simulink model "state_space_all_andres"  (R2018a)
settings: Solver=ode8  StartTime=0.0  StopTime=10  FixedStep=tm  RelTol=1e-3
InitFcn:
  | A_SimulinkInit_linea_transmision
values from neighbouring files (symbols this model uses):
  b = 4.91    [SimulinkInit_linea_transmision.m]
  C = 1    [SimulinkInit_linea_transmision.m]
  C1 = 22e-6    (= 2.2e-05)    [SimulinkInit_linea_transmision.m]
  C2 = 22e-6    (= 2.2e-05)    [SimulinkInit_linea_transmision.m]
  C3 = 610e-6    (= 0.00061)    [SimulinkInit_linea_transmision.m]
  Cl = 20000e-6    (= 0.02)    [SimulinkInit_linea_transmision.m]
  Jd = 0.3    [SimulinkInit_linea_transmision.m]
  K = 25    [SimulinkInit_linea_transmision.m]    (also in uio_linear.m = K1+E*H)
  K1 = 9.66    [SimulinkInit_linea_transmision.m]    (also in uio_linear.m = K1')
  K11 = 0.8    [SimulinkInit_linea_transmision.m]
  K1d = 1.15    [SimulinkInit_linea_transmision.m]
  K2 = 6.97    [SimulinkInit_linea_transmision.m]
  K22 = 0.2    [SimulinkInit_linea_transmision.m]
  K2d = 1    [SimulinkInit_linea_transmision.m]
  K3 = 31.8    [SimulinkInit_linea_transmision.m]
  K33 = 0.23    [SimulinkInit_linea_transmision.m]
  K3d = 1    [SimulinkInit_linea_transmision.m]
  K4 = 15.1    [SimulinkInit_linea_transmision.m]
  Kd = 0.02    [SimulinkInit_linea_transmision.m]
  Kdc = 0.02    [SimulinkInit_linea_transmision.m]
  Kf = 1    [SimulinkInit_linea_transmision.m]
  Kh = 1.2    [SimulinkInit_linea_transmision.m]
  Ks = 21.5    [SimulinkInit_linea_transmision.m]
  Ksc = 3    [SimulinkInit_linea_transmision.m]
  Kv = 1    [SimulinkInit_linea_transmision.m]
  L = 5.2    [SimulinkInit_linea_transmision.m]
  L1 = 40e-3    (= 0.04)    [SimulinkInit_linea_transmision.m]
  L2 = 30e-3    (= 0.03)    [SimulinkInit_linea_transmision.m]
  L3 = 5e-3    (= 0.005)    [SimulinkInit_linea_transmision.m]
  L4 = 35e-6    (= 3.5e-05)    [SimulinkInit_linea_transmision.m]
  L5 = 22e-6    (= 2.2e-05)    [SimulinkInit_linea_transmision.m]
  L6 = 10e-6    (= 1e-05)    [SimulinkInit_linea_transmision.m]
  Pd = 0.1    [SimulinkInit_linea_transmision.m]
  R = 10    [SimulinkInit_linea_transmision.m]
  R1 = 0.1    [SimulinkInit_linea_transmision.m]
  R2 = 0.2    [SimulinkInit_linea_transmision.m]
  R3 = 1e-3    (= 0.001)    [SimulinkInit_linea_transmision.m]
  R4 = 0.005    [SimulinkInit_linea_transmision.m]
  R5 = 0.0012    [SimulinkInit_linea_transmision.m]
  R6 = 0.001    [SimulinkInit_linea_transmision.m]
  RL = 10    [SimulinkInit_linea_transmision.m]
  Sbin = 13.8    [SimulinkInit_linea_transmision.m]
  Svin = 2.91    [SimulinkInit_linea_transmision.m]
  T1 = 0.4    [SimulinkInit_linea_transmision.m]
  T2 = 1    [SimulinkInit_linea_transmision.m]
  T3 = 15    [SimulinkInit_linea_transmision.m]
  T4 = 2.5    [SimulinkInit_linea_transmision.m]
  Tao1d = 0.5    [SimulinkInit_linea_transmision.m]
  Tao2d = 0.125    [SimulinkInit_linea_transmision.m]
  Tcd = 0.2    [SimulinkInit_linea_transmision.m]
  Tcr = 0.01    [SimulinkInit_linea_transmision.m]
  Tf = 0.04    [SimulinkInit_linea_transmision.m]
  Tr = 950    [SimulinkInit_linea_transmision.m]
  Tt = 450    [SimulinkInit_linea_transmision.m]
  Ttd = 0.04    [SimulinkInit_linea_transmision.m]
  Tv = 0.05    [SimulinkInit_linea_transmision.m]
  V = 20    [SimulinkInit_linea_transmision.m]
  wref = 70000    [SimulinkInit_linea_transmision.m]
  X_acid = 1.2    [SimulinkInit_linea_transmision.m]
  X_meth = 0.35    [SimulinkInit_linea_transmision.m]
  Z = 3    [SimulinkInit_linea_transmision.m]
undefined symbols (not defined in the file or in its folder): Ad, Bd, C1o, C2o, C3o, C4o, Cd, F1, F2, F3, F4, H1, H2, H3, H4, K1U, K2U, K3U, K4U, T1s, T2s, T3s, T4s, T5s, tm
libraries: dsparch4 x4, powerlib_meascontrol x4, mpclib x1, simulink x1
(part 1 of 2)
settings Model: Creator=MarioAndres  LastModifiedBy=MarioAndres

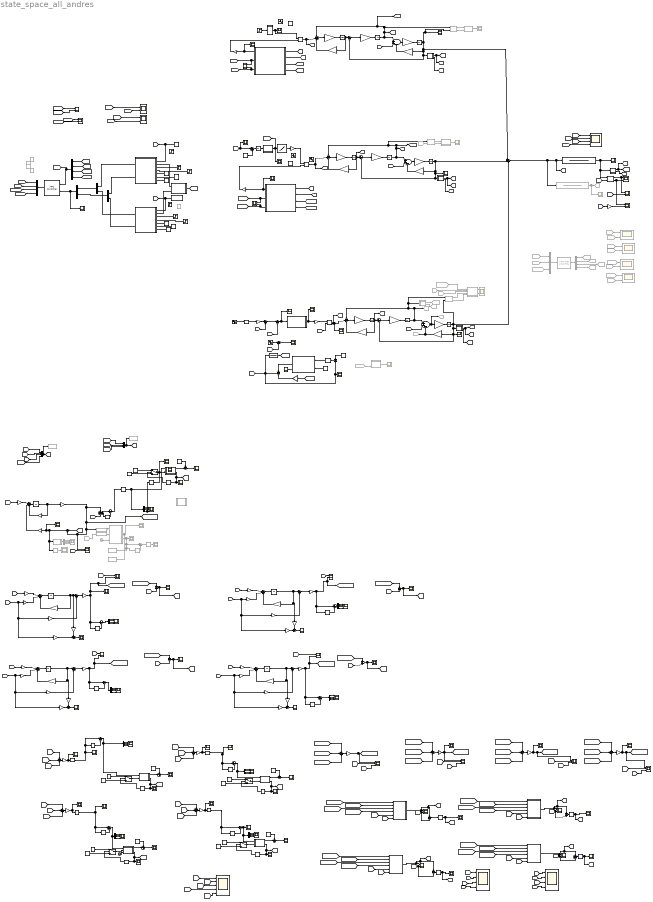
== system state_space_all_andres ==
  note: Nodo De Optimizacion
  note: CSI1-Biomasa
  note: CSI2-pv
  note: VSI-Diesel
  note: Carga RLC
  1-D Lookup Table2 : Lookup_n-D  NumberOfTableDimensions=1  BreakpointsForDimension1=[0 10 20 30 40 50 70 80 100]  Table=[0 10 200 500 800 1000 1140 1150 1200]  InternalRulePriority=Speed  RndMeth=Simplest  InputSameDT=on
  Abs{,1..3,5..9} (9 alike) : Abs
  Abs4 : Abs  Commented=on
  CSI_Control_BIO : Subsystem  mask{A=[0.0201   -0.039932     0.01986], B=[1     -1.9966       0.998], T=0.0001, st_time=0, Dn=[1     -1.0364], Dd=[1    -0.96364]}
      mask prompts: A "Numerador del control PR(z)"; B "Denominador del control PR(z)"; T "Tiempo de muestreo"; st_time "Tiempo_muerto"; Dn "Dn (Numerador de D(z))"; Dd "Dd (numerador de D(z))"
      mask DialogControl descripcion Prompt: Lazo de control de corriente para inversor monofasico. La entrada es un setpoint de potencia [P, Q]. Con ese setpoint se calcula la referencia de corriente sinusoidal deacuerdo a la tension medida de la red. Por lo anterior este controlador solo es valido para un inversor conectado a la red pues hara que se comporte como un CSI.
      mask DialogControl Control2 Prompt: Dn y Dd corresponden al numerador y denominador de la funcion de transferencia en Z (denominada D(z)) que hara un desfase de 90 de las señales medidas de tension y corriente del inversor. Estos desfases permiten mimificar las señales alfa y beta, de esta forma usar la misma teoria de potencia instantanea para el caso monofasico.
  CSI_Control_BIO1 : Subsystem  mask{A=[0.0201   -0.039932     0.01986], B=[1     -1.9966       0.998], T=0.0001, st_time=0, Dn=[1     -1.0364], Dd=[1    -0.96364]}
      mask prompts: A "Numerador del control PR(z)"; B "Denominador del control PR(z)"; T "Tiempo de muestreo"; st_time "Tiempo_muerto"; Dn "Dn (Numerador de D(z))"; Dd "Dd (numerador de D(z))"
      mask DialogControl descripcion Prompt: Lazo de control de corriente para inversor monofasico. La entrada es un setpoint de potencia [P, Q]. Con ese setpoint se calcula la referencia de corriente sinusoidal deacuerdo a la tension medida de la red. Por lo anterior este controlador solo es valido para un inversor conectado a la red pues hara que se comporte como un CSI.
      mask DialogControl Control2 Prompt: Dn y Dd corresponden al numerador y denominador de la funcion de transferencia en Z (denominada D(z)) que hara un desfase de 90 de las señales medidas de tension y corriente del inversor. Estos desfases permiten mimificar las señales alfa y beta, de esta forma usar la misma teoria de potencia instantanea para el caso monofasico.
  Clock1 : Clock  Commented=on
  Clock2 : Clock
  Constant : Constant  Commented=on  Value=-400
  Constant1 : Constant  Commented=on  Value=5000
  Constant{5..6,9..10,12,22..23,27..28,32} (10 alike) : Constant
  Constant11 : Constant  Value=1000
  Constant13 : Constant  Value=6000
  Constant14 : Constant  Value=5000
  Constant15 : Constant  Value=972.8
  Constant16 : Constant  Value=8000
  Constant17 : Constant  Value=115400
  Constant18 : Constant  Value=5000
  Constant19 : Constant  Value=8000
  Constant2 : Constant  Commented=on  Value=5000
  Constant20 : Constant  Value=10000
  Constant{7..8,21,24,31} (5 alike) : Constant  Value=0
  Constant25 : Constant  Value=1000
  Constant26 : Constant  Commented=on  Value=11210
  Constant29 : Constant  Value=1000
  Constant3 : Constant  Commented=on  Value=8000
  Constant30 : Constant  Value=0.1
  Control PR VSI1 : Subsystem
  Current Panel : Constant  Value=1.5
  Delay : Delay  DelayLength=1
  Demux : Demux  Commented=on
  Demux{1..4,9..14} (10 alike) : Demux
  Demux19 : Demux  Commented=on
  Derivative2 : Derivative  CoefficientInTFapproximation=0
  Derivative4 : Derivative  Commented=on  CoefficientInTFapproximation=0
  Diesel Generator2 : Subsystem
  From : From  Commented=on  GotoTag=i1model
  From14 : From  Commented=on  GotoTag=i1
  From15 : From  Commented=on  GotoTag=i2
  From24 : From  Commented=on  GotoTag=Vload
  From25 : From  Commented=on  GotoTag=i3
  From30 : From  Commented=on  GotoTag=u2
  From33 : From  Commented=on  GotoTag=u3
  From37 : From  Commented=on  GotoTag=Papadiel
  From38 : From  Commented=on  GotoTag=Paparente
  From39 : From  Commented=on  GotoTag=Q_ref
  From40 : From  Commented=on  GotoTag=P_ref
  From47 : From  Commented=on  GotoTag=i2
  From6 : From  Commented=on  GotoTag=i2model
  From60 : From  Commented=on  GotoTag=y_ma
  From7 : From  Commented=on  GotoTag=i3model
  From8 : From  Commented=on  GotoTag=Vloadm
  From9 : From  Commented=on  GotoTag=u1
  Gain : Gain  Gain=1/L1
  Gain1 : Gain  Gain=1/C1
  Gain10 : Gain  Gain=1/L3
  Gain11 : Gain  Gain=1/C3
  Gain12 : Gain  Gain=1/L6
  Gain13 : Gain  Gain=R6
  Gain14 : Gain  Gain=R3
  Gain{15..18} (4 alike) : Gain  Gain=2
  Gain19 : Gain  Gain=C3
  Gain2 : Gain  Gain=1/L4
  Gain20 : Gain  Gain=-1
  Gain21 : Gain  Gain=.5
  Gain{22..29} (8 alike) : Gain  Gain=1/3
  Gain3 : Gain  Gain=R4
  Gain4 : Gain  Gain=R1
  Gain5 : Gain  Gain=1/L2
  Gain6 : Gain  Gain=1/C2
  Gain7 : Gain  Gain=1/L5
  Gain8 : Gain  Gain=R5
  Gain9 : Gain  Gain=R2
  Goto : Goto  Commented=on  GotoTag=i1model
  Goto1 : Goto  Commented=on  GotoTag=Vload
  Goto15 : Goto  Commented=on  GotoTag=i2model
  Goto16 : Goto  Commented=on  GotoTag=i3model
  Goto17 : Goto  Commented=on  GotoTag=v3
  Goto18 : Goto  Commented=on  GotoTag=vl6
  Goto19 : Goto  Commented=on  GotoTag=vr6
  Goto22 : Goto  Commented=on  GotoTag=Vloadm
  Goto61 : Goto  Commented=on  GotoTag=V_vsi
  Goto62 : Goto  Commented=on  GotoTag=a4
  Integrator{,1..8} (9 alike) : Integrator
  Integrator9 : Integrator  LimitOutput=on  UpperSaturationLimit=1  LowerSaturationLimit=0
  LinearProg2 : MATLAB Function  TreatAsAtomicUnit=on  SystemSampleTime=1e-3
  LinearProg3 : MATLAB Function  TreatAsAtomicUnit=on  SystemSampleTime=1e-3
  MATLAB Funcionando sin Vload conectado despues del ataque : MATLAB Function  Commented=on  TreatAsAtomicUnit=on
  "MATLAB Function SOC " : MATLAB Function  TreatAsAtomicUnit=on
  MATLAB Function1 : MATLAB Function  TreatAsAtomicUnit=on
  MATLAB Function12 : MATLAB Function  TreatAsAtomicUnit=on
  MATLAB Function13 : MATLAB Function  TreatAsAtomicUnit=on
  MATLAB Function17 : MATLAB Function  TreatAsAtomicUnit=on
  MATLAB Function18 : MATLAB Function  TreatAsAtomicUnit=on
  MATLAB Function2 : MATLAB Function  TreatAsAtomicUnit=on
  MATLAB Function3 : MATLAB Function  Commented=on  TreatAsAtomicUnit=on
  MATLAB Function34 : MATLAB Function  TreatAsAtomicUnit=on
  MATLAB Function36 : MATLAB Function  TreatAsAtomicUnit=on
  MATLAB Function38 : MATLAB Function  TreatAsAtomicUnit=on
  MATLAB Function39 : MATLAB Function  TreatAsAtomicUnit=on
  MATLAB Function4 : MATLAB Function  Commented=on  TreatAsAtomicUnit=on
  MATLAB Function5 : MATLAB Function  Commented=on  TreatAsAtomicUnit=on
  MATLAB Function6 : MATLAB Function  Commented=on  TreatAsAtomicUnit=on
  MATLAB Function7 : MATLAB Function  Commented=on  TreatAsAtomicUnit=on
  MATLAB Function8 : MATLAB Function  Commented=on  TreatAsAtomicUnit=on
  MPC Controller : mpclib/MPC Controller  SCDEnableBlockLinearizationSpecification=on  mpcobj=mpcobj  is_multiple=0  enable_value=0  return_u0=off  updateMPCinCallerWorkspace=on  ref_from_ws=off  ref_signal_name=[]  ref_preview=off  md_from_ws=off  md_signal_name=[]  md_preview=off  from_project=off  project_file=MPCtask.mat  md_inport=off  mv_inport=off  cost_outport=off  return_sequence=off  return_qpstatus=off  return_state=off  state_inport=off  lims_inport=off  cc_inport=off  ywt_inport=off  is_designfromscratch=0  uwt_inport=off  duwt_inport=off  rhoeps_inport=off  uref_inport=off  n_ts=0.1  n_p=100  n_mv=4  n_md=0  n_ud=0  n_mo=4  n_uo=0  BlockDataType=double  SampleTimeInherited=off  switch_inport=off
  MeasureNode_I1 : Subsystem
  MeasureNode_I2 : Subsystem
  MeasureNode_I3 : Subsystem
  MeasureNode_I4 : Subsystem
  MeasureNode_I5 : Subsystem  Commented=on
  Memory{,1..13} (14 alike) : Memory
  Memory14 : Memory  Commented=on
  Mux2 : Mux  Commented=on  Inputs=3
  Mux3 : Mux  Inputs=2
  Mux4 : Mux
  Mux5 : Mux  Inputs=2
  Mux6 : Mux  Inputs=2
  Mux7 : Mux  Inputs=3
  Mux8 : Mux
  PID Controller2 : simulink/Continuous/PID Controller  Controller=PID  TimeDomain=Continuous-time  SampleTime=-1  IntegratorMethod=Forward Euler  FilterMethod=Forward Euler  Form=Parallel  UseFilter=on  ControllerParametersSource=internal  P=0.000853612192208084  I=3.94394231511782e-05  D=0.00224356290205903  N=0.155980576752107  InitialConditionSource=internal  InitialConditionForIntegrator=0  InitialConditionForFilter=0  ExternalReset=none  LimitOutput=off  UpperSaturationLimit=inf  LowerSaturationLimit=-inf  LinearizeAsGain=on  AntiWindupMode=none  Kb=1  TrackingMode=off  Kt=1  PParamMin=[]  PParamMax=[]  IParamMin=[]  IParamMax=[]  DParamMin=[]  DParamMax=[]  NParamMin=[]  NParamMax=[]  KbParamMin=[]  KbParamMax=[]  KtParamMin=[]  KtParamMax=[]  POutMin=[]  POutMax=[]  IOutMin=[]  IOutMax=[]  DOutMin=[]  DOutMax=[]  NOutMin=[]  NOutMax=[]  KbOutMin=[]  KbOutMax=[]  KtOutMin=[]  KtOutMax=[]  IntegratorOutMin=[]  IntegratorOutMax=[]  FilterOutMin=[]  FilterOutMax=[]  SumOutMin=[]  SumOutMax=[]  SumI1OutMin=[]  SumI1OutMax=[]  SumI2OutMin=[]  SumI2OutMax=[]  SumI3OutMin=[]  SumI3OutMax=[]  SumDOutMin=[]  SumDOutMax=[]  SaturationOutMin=[]  SaturationOutMax=[]  IntegratorContinuousStateAttributes=''  IntegratorStateMustResolveToSignalObject=off  IntegratorRTWStateStorageClass=Auto  FilterContinuousStateAttributes=''  FilterStateMustResolveToSignalObject=off  FilterRTWStateStorageClass=Auto  DifferentiatorICPrevScaledInput=0  DifferentiatorOutMin=[]  DifferentiatorOutMax=[]  InitialConditionSetting=State (most efficient)  FilterDiffOutCoefMin=[]  FilterDiffOutCoefMax=[]  SumDenOutMin=[]  SumDenOutMax=[]  SumNumOutMin=[]  SumNumOutMax=[]  ReciprocalOutMin=[]  ReciprocalOutMax=[]  DivideOutMin=[]  DivideOutMax=[]  TunerSelectOption=Transfer Function Based (PID Tuner App)
  Power : powerlib_meascontrol/Measurements/Power  Freq=60  Vinit=[1, 0]  Iinit=[1, 0]  Ts=0
      settings: SourceProductName=Simscape Power Systems
  Power1 : powerlib_meascontrol/Measurements/Power  Commented=on  Freq=60  Vinit=[1, 0]  Iinit=[1, 0]  Ts=0
      settings: SourceProductName=Simscape Power Systems
  Power3 : powerlib_meascontrol/Measurements/Power  Commented=on  Freq=60  Vinit=[1, 0]  Iinit=[1, 0]  Ts=0
      settings: SourceProductName=Simscape Power Systems
  Power4 : powerlib_meascontrol/Measurements/Power  Commented=on  Freq=60  Vinit=[1, 0]  Iinit=[1, 0]  Ts=0
      settings: SourceProductName=Simscape Power Systems
  Product : Product
  Product1 : Product
  Product3 : Product
  Scope{,1,3,7,35} (5 alike) : Scope  Commented=on  NumInputPorts=2
  Scope{8,10..12,14..18,21,52..53,58,86..89,109} (18 alike) : Scope  NumInputPorts=2
  Scope{2,4..6,13,19..20,24..32,34,37..38,41..49,51,55..57,61,63..73,75,91,110,112,114,118,120..121,135} (53 alike) : Scope
  Scope{59..60,62,138} (4 alike) : Scope  NumInputPorts=3
  Scope{9,22,36,39..40,50,74,139} (8 alike) : Scope  Commented=on
  Scope{23,33,76..83,85,90} (12 alike) : Scope  NumInputPorts=4
  Scope54 : Scope  Commented=on  NumInputPorts=4
  Scope84 : Scope  NumInputPorts=5
  Signal Specification : SignalSpecification  Commented=on  Dimensions=4
  Signal Specification1 : SignalSpecification  Commented=on  Dimensions=4
  Sine Wave1 : Sin  Amplitude=170  Frequency=2*pi*60  SampleTime=0
  Sine Wave2 : Sin  Frequency=2*pi/0.025  SampleTime=0
  Sine Wave3 : Sin  Frequency=2*pi/0.025  SampleTime=0
  Sine Wave4 : Sin  Amplitude=170  Frequency=2*pi*60  SampleTime=0
  Sine Wave5 : Sin  Amplitude=60  Frequency=2*pi*60  SampleTime=0
  State-Space : StateSpace  Commented=on  A=|  B=|  C=[zeros(1,3) 1 zeros(1,7); zeros(1,4) 1 zeros(1,6); zeros(1,5) 1 zeros(1,5);zeros(1,10) 1]  D=zeros(4,3);  InitialCondition=0
      A=|
      | [-R1/L1 zeros(1,6) -1/L1 zeros(1,3);
      |     0 -R2/L2 zeros(1,6) -1/L2 0 0;
      |     zeros(1,2) -R3/L3 zeros(1,6) -1/L3 0;
      |     zeros(1,3) -R4/L4 zeros(1,3) 1/L4 0 0 -1/L4;
      |     zeros(1,4) -R5/L5 zeros(1,3) 1/L5 0 -1/L5;
      |     zeros(1,5) -R6/L6 zeros(1,3) 1/L6 -1/L6;
      |     zeros(1,6) -R/L zeros(1,3) 1/L;
      |     1/C1 zeros(1,2) -1/C1 zeros(1,7);
      |     0 1/C2 0 0 -1/C2 zeros(1,6);
      |     0 0 1/C3 0 0 -1/C3 zeros(1,5);
      |     zeros(1,3) 1/Cl 1/Cl 1/Cl -1/Cl zeros(1,3) -1/(Cl*RL)]
      B=|
      | [1/L1 0 0;
      |    0 1/L2 0;
      |    0 0 1/L3;
      |    zeros(8,3)];
  Step : Step  Time=0  After=28  SampleTime=0
  Step1 : Step  Time=200  Before=1.2  After=.4  SampleTime=0
  Step10 : Step  Time=20  Before=115400  After=15400  SampleTime=0
  Step4 : Step  Time=200  Before=1  After=0.4  SampleTime=0
  Step5 : Step  Time=200  Before=1  SampleTime=0
  Step8 : Step  Time=200  Before=.7  SampleTime=0
  Step9 : Step  Time=20  Before=978  After=1400  SampleTime=0
  Sum{,4,7,11,17,20,24..26,30,36..37,39..40,43} (15 alike) : Sum  Inputs=|+-
  Sum1 : Sum  Inputs=|+--
  Sum{10,12,14,22,38,74} (6 alike) : Sum  Inputs=|++
  Sum{13,15..16,18,27,33,42,67,70,72..73} (11 alike) : Sum  Inputs=+-
  Sum{19,31..32,71} (4 alike) : Sum  Inputs=-+|
  Sum2 : Sum  Inputs=|+++
  Sum{21,23,49,75..76} (5 alike) : Sum  Inputs=|+++  SampleTime=tm
  Sum{28..29,34..35,53} (5 alike) : Sum  Inputs=+-|
  Sum3 : Sum  Inputs=-|+-
  Sum41 : Sum  Commented=on  Inputs=|+-
  Sum5 : Sum  Inputs=|+--
  Sum{58..61,77..80} (8 alike) : Sum  Inputs=+++
  Sum6 : Sum  Inputs=-|+-
  Sum8 : Sum  Inputs=|+--
  Sum9 : Sum  Inputs=-|+-
  Switch{,1..4} (5 alike) : Switch  Criteria=u2 > Threshold
  To Workspace : ToWorkspace  Commented=on  VariableName=det1  SampleTime=1e-4
  To Workspace1 : ToWorkspace  Commented=on  VariableName=norm1  SampleTime=1e-4
  To Workspace2 : ToWorkspace  Commented=on  VariableName=y_ma  SampleTime=1e-4
  To Workspace3 : ToWorkspace  Commented=on  VariableName=u_fs  SampleTime=1e-4
  Transfer Fcn1 : TransferFcn  Commented=on  Numerator=[R*RL*L 0]  Denominator=[Cl*RL*R*L (RL+R)*L R*RL]
  Transfer Fcn3 : TransferFcn  Numerator=[RL*L RL*R]  Denominator="[Cl*RL*L  (R*RL*Cl+L) RL+R]"
  Transfer Fcn4 : TransferFcn  Denominator=[1e-4 1]
  Unit Delay{1..2,6..7,10} (5 alike) : UnitDelay  SampleTime=tm
  adis1 : Gain  Gain=F3  Multiplication=Matrix(K*u) (u vector)  SampleTime=tm
  adis10 : Gain  Gain=Ld'  Multiplication=Matrix(K*u) (u vector)  SampleTime=tm
  adis11 : Gain  Gain=F1  Multiplication=Matrix(K*u) (u vector)  SampleTime=tm
  adis12 : Gain  Gain=F2  Multiplication=Matrix(K*u) (u vector)  SampleTime=tm
  adis2 : Gain  Gain=F4  Multiplication=Matrix(K*u) (u vector)  SampleTime=tm
  adis7 : Gain  Gain=Ad  Multiplication=Matrix(K*u) (u vector)  SampleTime=tm
  bdis1 : Gain  Gain=T3*Bd  Multiplication=Matrix(K*u) (u vector)  SampleTime=tm
  bdis10 : Gain  Gain=T2*Bd  Multiplication=Matrix(K*u) (u vector)  SampleTime=tm
  bdis11 : Gain  Gain=K2U  Multiplication=Matrix(K*u) (u vector)  SampleTime=tm
  bdis12 : Gain  Gain=H2  Multiplication=Matrix(K*u) (u vector)  SampleTime=tm
  bdis13 : Gain  Gain=eye(1)-C2o*H2  Multiplication=Matrix(K*u) (u vector)  SampleTime=tm
  bdis14 : Gain  Gain=eye(1)-C1o*H1  Multiplication=Matrix(K*u) (u vector)  SampleTime=tm
  bdis15 : Gain  Gain=C1o  Multiplication=Matrix(K*u) (u vector)  SampleTime=tm
  bdis16 : Gain  Gain=C2o  Multiplication=Matrix(K*u) (u vector)  SampleTime=tm
  bdis17 : Gain  Gain=T4*Bd  Multiplication=Matrix(K*u) (u vector)  SampleTime=tm
  bdis18 : Gain  Gain=K4U  Multiplication=Matrix(K*u) (u vector)  SampleTime=tm
  bdis19 : Gain  Gain=H4  Multiplication=Matrix(K*u) (u vector)  SampleTime=tm
  bdis2 : Gain  Gain=K3U  Multiplication=Matrix(K*u) (u vector)  SampleTime=tm
  bdis20 : Gain  Gain=eye(1)-C4o*H4  Multiplication=Matrix(K*u) (u vector)  SampleTime=tm
  bdis21 : Gain  Gain=C4o  Multiplication=Matrix(K*u) (u vector)  SampleTime=tm
  bdis3 : Gain  Gain=H3  Multiplication=Matrix(K*u) (u vector)  SampleTime=tm
  bdis4 : Gain  Gain=eye(1)-C3o*H3  Multiplication=Matrix(K*u) (u vector)  SampleTime=tm
  bdis5 : Gain  Gain=Bd  Multiplication=Matrix(K*u) (u vector)  SampleTime=tm
  bdis6 : Gain  Gain=C3o  Multiplication=Matrix(K*u) (u vector)  SampleTime=tm
  bdis7 : Gain  Gain=T1*Bd  Multiplication=Matrix(K*u) (u vector)  SampleTime=tm
  bdis8 : Gain  Gain=K1U  Multiplication=Matrix(K*u) (u vector)  SampleTime=tm
  bdis9 : Gain  Gain=H1  Multiplication=Matrix(K*u) (u vector)  SampleTime=tm
  cdis{1..5} (5 alike) : Gain  Gain=Cd  Multiplication=Matrix(K*u) (u vector)  SampleTime=tm
  generador biomasa : Subsystem
  wires:
  Gain/1 -> Integrator/1
  Integrator/1 -> Gain4/1, Sum/1
  Sum/1 -> Gain1/1
  Gain1/1 -> Integrator1/1
  Integrator1/1 -> [v1], [V_bio], Sum3/1, Power3/1, Sum1/1
  Sum1/1 -> Gain2/1
  Gain2/1 -> Integrator2/1
  Integrator2/1 -> Power3/2, Scope4/1, Sum2/1, MeasureNode_I2/1(in), Sum/2, Gain3/1
  Gain3/1 -> Sum1/3
  Sum3/1 -> Gain/1
  Gain4/1 -> Sum3/3
  Sum2/1 -> Transfer Fcn1/1, [I_load], Transfer Fcn3/1
  Transfer Fcn3/1 -> MeasureNode_I4/1(in), Power/1, Scope2/1
  [Vload] -> Sum1/2
  Integrator3/1 -> [ipi], Gain9/1, Sum4/1
  Gain5/1 -> Integrator3/1
  Gain6/1 -> Integrator4/1
  Gain8/1 -> Sum5/3
  Gain7/1 -> Integrator5/1
  [Vload] -> Sum5/2
  Gain9/1 -> Sum6/3
  Sum6/1 -> Gain5/1
  Sum5/1 -> Gain7/1
  Sum4/1 -> Gain6/1
  Integrator6/1 -> [i3m], Gain14/1, Sum7/1
  Gain10/1 -> Integrator6/1
  Gain11/1 -> Integrator7/1
  Integrator7/1 -> MeasureNode_I5/1(in), Power1/1, Sum9/1, Goto17/1, Sum8/1
  Gain13/1 -> Goto19/1, Sum8/3
  Gain12/1 -> Integrator8/1
  [Vload] -> Sum8/2
  Gain14/1 -> Sum9/3
  Sum9/1 -> Gain10/1
  Sum8/1 -> Goto18/1, Gain12/1
  Sum7/1 -> Gain11/1
  Integrator8/1 -> Power1/2, Sum2/3, MeasureNode_I3/1(in), Gain13/1, Scope6/1, Sum7/2
  Integrator5/1 -> Sum2/2, Scope5/1, MeasureNode_I1/1(in), Sum4/2, Gain8/1
  [I_load] -> Power/2
  Power/1 -> Scope11/1, Scope10/1
  Power/2 -> Scope12/1, Scope10/2
  [P_ref] -> Scope11/2
  CSI_Control_BIO/2(Q_measure) -> [Qo_bio], Scope14/1
  CSI_Control_BIO/3(P_measure) -> [Po_bio], Scope14/2
  Control PR VSI1/1(d) -> Gain17/1, Scope28/1
  Product3/1 -> [u3], Sum9/2, Scope29/1
  CSI_Control_BIO1/2(Q_measure) -> [Qo_diesel], Scope21/1
  CSI_Control_BIO1/3(P_measure) -> [Po_diesel], Scope21/2
  Integrator4/1 -> [v2], [V_die], Power4/1, Sum6/1, Sum5/1
  Current Panel/1 -> Sum14/2
  Sum14/1 -> Integrator9/1
  [ipi] -> Scope27/1, Sum14/1  "inductor I measured"
  "MATLAB Function SOC "/1(y) -> [SOC], Scope26/1, 1-D Lookup Table2/1  "soc"
  1-D Lookup Table2/1 -> Gain18/1  "battery Vdc"
  Integrator9/1 -> "MATLAB Function SOC "/1(u)
  Derivative2/1 -> Gain19/1
  Gain19/1 -> Sum12/1
  Sine Wave1/1 -> Derivative2/1  "ref voltage"
  Sum11/1 -> Control PR VSI1/1(Ierror), Scope19/1
  Sum12/1 -> Sum11/1
  [i3] -> Sum12/2
  [i3m] -> Sum11/2
  Product1/1 -> Sum6/2, [u2]
  Step5/1 -> LinearProg3/3(kb)
  Mux4/1 -> [Paparente], MPC Controller/1
  Constant13/1 -> LinearProg3/7(Q_e_alt_min)
  [Qo_bio] -> Mux4/2
  Mux3/1 -> Scope32/1, MPC Controller/2
  LinearProg2/2(Pdo) -> Mux6/1  "die"
  Mux6/1 -> Mux3/2
  [SOC] -> MATLAB Function2/1(SOC)
  MPC Controller/1 -> Demux3/1
  [Qo_diesel] -> Mux4/4
  Constant14/1 -> LinearProg3/6(QbMax)
  Constant18/1 -> LinearProg2/7(P_e_alt_min)
  Mux5/1 -> Mux3/1
  [Po_diesel] -> Mux4/3
  Step4/1 -> LinearProg2/4(kd)
  Step1/1 -> LinearProg2/3(kb)
  Constant19/1 -> LinearProg3/5(QdMax)
  MATLAB Function2/1(MaxP) -> LinearProg2/2(P_e_alt)
  Constant20/1 -> LinearProg2/6(PbMax)
  MATLAB Function2/2(MaxQ) -> LinearProg3/2(Q_e_alt)
  Step8/1 -> LinearProg3/4(kd)
  LinearProg3/2(Qdo) -> Mux6/2
  [Po_bio] -> Mux4/1
  LinearProg3/1(Qbo) -> Mux5/2
  Constant16/1 -> LinearProg2/5(PdMax)
  LinearProg2/1(Pbo) -> Mux5/1  "bio"
  [Pi_bio] -> Scope16/2
  [Po_bio] -> Scope16/1
  [Qi_bio] -> Scope15/2
  [Qo_bio] -> Scope15/1
  [Qo_diesel] -> Scope17/1
  [Po_diesel] -> Scope18/1
  [Pi_Diesel] -> Scope18/2
  [Qi_diesel] -> Scope17/2
  [V_vsi] -> Scope23/4
  [V_die] -> Scope23/3
  [V_bio] -> Scope23/2
  [Vload] -> Scope23/1
  generador biomasa/1(Vdc) -> Product/1, Scope24/1
  Step/1 -> generador biomasa/1(In1)
  [v2] -> CSI_Control_BIO1/1(V_measured)
  [i2] -> CSI_Control_BIO1/2(I_measured)
  [v1] -> CSI_Control_BIO/1(V_measured)
  [i1] -> CSI_Control_BIO/2(I_measured)
  Gain18/1 -> Product1/1
  Gain15/1 -> Product/2
  Product/1 -> [u1], Sum3/2
  Gain16/1 -> Product1/2
  [Pi_Diesel] -> CSI_Control_BIO1/3(P_ref)
  [Qi_diesel] -> CSI_Control_BIO1/4(Q_ref)
  Gain17/1 -> Product3/1
  [Pi_bio] -> CSI_Control_BIO/3(P_ref)
  [Qi_bio] -> CSI_Control_BIO/4(Q_ref)
  [Q_ref] -> Gain20/1
  Gain20/1 -> Scope12/2
  MATLAB Function3/1(y) -> Scope22/1
  From37/1 -> MATLAB Function3/3(potencia)
  From38/1 -> MATLAB Function4/1(u)
  From40/1 -> MATLAB Function4/2(pref)
  From39/1 -> MATLAB Function4/3(qref)
  Power1/1 -> MATLAB Function4/4(pm)
  Power1/2 -> MATLAB Function4/5(qm)
  MATLAB Function4/1(y) -> Scope35/1
  MATLAB Function4/2(pam) -> Scope35/2
  Constant30/1 -> Diesel Generator2/2(Par de Carga)
  Transfer Fcn4/1 -> [Io_diesel]
  Sum13/1 -> PID Controller2/1
  [Io_diesel] -> Gain21/1
  Gain21/1 -> Sum15/2
  PID Controller2/1 -> Diesel Generator2/1(in)
  Sum15/1 -> [Vdc], Scope37/1, Sum13/2, Transfer Fcn4/1  "Output DC Voltage"
  Constant29/1 -> Sum13/1
  Diesel Generator2/2(Power) -> Sum15/1
  Diesel Generator2/3(caudal) -> Scope38/1
  [Vdc] -> Product3/2
  Power3/1 -> MATLAB Function5/1(p)
  Power3/2 -> MATLAB Function5/2(q)
  MATLAB Function5/1(y) -> Scope39/1
  Power4/2 -> MATLAB Function6/2(q)
  Power4/1 -> MATLAB Function6/1(p)
  MATLAB Function6/1(y) -> Scope40/1
  From47/1 -> Power4/2
  From9/1 -> Mux2/1
  From30/1 -> Mux2/2
  From33/1 -> Mux2/3
  Mux2/1 -> State-Space/1
  State-Space/1 -> Demux/1
  Demux/1 -> Goto/1
  Demux/2 -> Goto15/1
  Demux/3 -> Goto16/1
  Demux/4 -> Goto22/1
  From14/1 -> Scope/1
  From/1 -> Scope/2
  From15/1 -> Scope1/1
  From6/1 -> Scope1/2
  From25/1 -> Scope3/1
  From7/1 -> Scope3/2
  From24/1 -> Scope7/1
  From8/1 -> Scope7/2
  Demux3/4 -> [Qi_diesel]
  Demux3/3 -> [Pi_Diesel]
  Demux3/2 -> [Qi_bio]
  Demux3/1 -> [Pi_bio]
  cdis4/1 -> Sum33/1, [x_hat], Signal Specification/1, Scope8/1, Sum17/2
  [V_vsi] -> Mux8/4
  MATLAB Function7/1(y) -> Demux19/1
  Sum17/1 -> Derivative4/1, MATLAB Function7/1(r), Scope48/1, adis10/1
  Mux7/1 -> To Workspace3/1, [u_fs]
  MATLAB Function8/2(norm_rd) -> Sum41/1, Memory14/1, To Workspace1/1, Scope50/1
  Clock1/1 -> MATLAB Function8/3(tiempo)
  bdis5/1 -> Sum75/1
  Signal Specification/1 -> MATLAB Function8/1(y_hat)
  Demux19/2 -> Scope54/2
  [y_ma] -> Sum17/1
  [I3] -> Mux8/3
  [I2] -> Mux8/2
  [u_fs] -> bdis5/1
  Mux8/1 -> To Workspace2/1, [y_ma]
  Derivative4/1 -> Scope139/1
  Signal Specification1/1 -> MATLAB Function8/2(y_m)
  adis7/1 -> Sum75/3
  From60/1 -> Signal Specification1/1
  Unit Delay6/1 -> cdis4/1, adis7/1
  adis10/1 -> Sum75/2
  Sum75/1 -> Unit Delay6/1
  [I1] -> Mux8/1
  Demux19/1 -> Scope54/1
  Demux19/3 -> Scope54/3
  Demux19/4 -> Scope54/4
  [u1] -> Mux7/1
  [u2] -> Mux7/2
  [u3] -> Mux7/3
  [y_ma] -> Scope8/2
  MeasureNode_I2/1(Out) -> [i1], [I1]
  MATLAB Function8/1(rol) -> To Workspace/1, Scope9/1
  bdis9/1 -> Sum10/2
  bdis11/1 -> Sum23/2
  Unit Delay7/1 -> adis11/1, bdis15/1, Sum10/1
  adis12/1 -> Sum23/3
  bdis21/1 -> Sum19/1
  Sum31/1 -> Scope65/1
  [I2] -> bdis14/1, bdis9/1, bdis8/1
  [y_ma] -> Scope86/1
  [u_fs] -> bdis1/1
  [y_ma] -> Scope88/1
  adis11/1 -> Sum21/3
  Sum76/1 -> Unit Delay2/1
  bdis14/1 -> Sum31/2
  bdis12/1 -> Sum22/2
  Unit Delay10/1 -> bdis16/1, adis12/1, Sum22/1
  bdis3/1 -> Sum38/2
  Sum32/1 -> Scope66/1
  [I3] -> bdis13/1, bdis12/1, bdis11/1
  Unit Delay2/1 -> bdis21/1, adis2/1, Sum74/1
  bdis4/1 -> Sum71/2
  bdis2/1 -> Sum49/2
  [y_ma] -> Scope89/1
  Unit Delay1/1 -> bdis6/1, adis1/1, Sum38/1
  adis1/1 -> Sum49/3
  Sum10/1 -> cdis1/1
  bdis10/1 -> Sum23/1
  [u_fs] -> bdis7/1
  bdis17/1 -> Sum76/1
  bdis18/1 -> Sum76/2
  [u_fs] -> bdis10/1
  bdis13/1 -> Sum32/2
  Sum21/1 -> Unit Delay7/1
  bdis6/1 -> Sum71/1
  bdis7/1 -> Sum21/1
  Sum19/1 -> Scope72/1
  bdis20/1 -> Sum19/2
  bdis1/1 -> Sum49/1
  bdis16/1 -> Sum32/1
  adis2/1 -> Sum76/3
  [V_vsi] -> bdis4/1, bdis3/1, bdis2/1
  bdis15/1 -> Sum31/1
  Sum49/1 -> Unit Delay1/1
  [I1] -> bdis20/1, bdis19/1, bdis18/1
  [y_ma] -> Scope87/1
  Sum22/1 -> cdis2/1
  bdis19/1 -> Sum74/2
  Sum74/1 -> cdis5/1
  Sum71/1 -> Scope67/1
  Sum23/1 -> Unit Delay10/1
  [u_fs] -> bdis17/1
  bdis8/1 -> Sum21/2
  cdis1/1 -> Memory10/1, Sum36/1, [x_hat_uio11], Scope86/2, Scope61/1
  Sum38/1 -> cdis3/1
  cdis3/1 -> Memory12/1, Sum39/1, Scope88/2, [x_hat_uio13]
  cdis5/1 -> Memory13/1, Sum40/1, [x_hat_uio21], Scope89/2
  [x_hat_uio21] -> Sum67/1
  [y_ma] -> Sum67/2
  [x_hat_uio11] -> Sum70/1
  [y_ma] -> Sum70/2
  [x_hat_uio12] -> Sum72/1
  [y_ma] -> Sum72/2
  [x_hat_uio13] -> Sum73/1
  [y_ma] -> Sum73/2
  [druo3] -> Sum77/3
  [druo2] -> Sum77/2
  Sum77/1 -> Gain22/1
  [druo1] -> Sum77/1
  Gain22/1 -> Abs/1, Scope110/1
  Sum78/1 -> Gain23/1
  [druo3] -> Sum78/2
  [druo2] -> Sum78/1
  [druo4] -> Sum78/3
  [druo4] -> Sum79/3
  Sum79/1 -> Gain24/1
  [druo1] -> Sum79/2
  [druo3] -> Sum79/1
  [druo1] -> Sum80/3
  Sum80/1 -> Gain25/1
  [druo2] -> Sum80/2
  [druo4] -> Sum80/1
  Gain23/1 -> Abs2/1, Scope112/1
  Gain25/1 -> Scope118/1, Abs3/1
  Gain24/1 -> Abs1/1, Scope114/1
  MeasureNode_I1/1(Out) -> [i2], [I2]
  MeasureNode_I3/1(Out) -> [I3], [i3]
  Sum70/1 -> [druo1], Scope30/1
  Sum72/1 -> [druo2], Scope43/1
  Sum73/1 -> [druo3], Scope44/1
  Sum67/1 -> [druo4], Scope45/1
  Memory/1 -> Sum20/2
  Constant8/1 -> Switch/1
  Sum20/1 -> Demux10/1, MATLAB Function36/1(dr)
  MATLAB Function36/1(r) -> Sum53/2
  MATLAB Function36/2(c) -> [ruo1], Scope121/1, Memory1/1
  Switch/1 -> MATLAB Function36/2(ban)
  Sum53/1 -> Scope120/1
  Memory1/1 -> Switch/2
  Constant9/1 -> Switch/3
  Constant5/1 -> Sum53/1
  Memory2/1 -> Sum24/2
  Memory3/1 -> Sum25/2
  Sum25/1 -> Demux12/1, MATLAB Function17/1(dr)
  Memory4/1 -> Sum26/2
  Sum26/1 -> Demux13/1, MATLAB Function18/1(dr), Scope46/1
  Constant6/1 -> Sum28/1
  Constant10/1 -> Switch1/3
  Switch1/1 -> MATLAB Function17/2(ban)
  MATLAB Function17/2(c) -> [ruo2], Scope49/1, Memory5/1
  Memory5/1 -> Switch1/2
  Sum28/1 -> Scope47/1
  Constant7/1 -> Switch1/1
  MATLAB Function17/1(r) -> Sum28/2
  Constant12/1 -> Sum29/1
  Constant22/1 -> Switch2/3
  Switch2/1 -> MATLAB Function18/2(ban)
  MATLAB Function18/2(c) -> [ruo4], Scope56/1, Memory6/1
  Memory6/1 -> Switch2/2
  Sum29/1 -> Scope55/1
  Constant21/1 -> Switch2/1
  MATLAB Function18/1(r) -> Sum29/2
  Memory7/1 -> Sum30/2
  [y_ma] -> Sum33/2
  Sum33/1 -> Sum30/1, Memory7/1
  Constant23/1 -> Sum34/1
  Constant27/1 -> Switch3/3
  Switch3/1 -> Scope75/1, MATLAB Function12/2(ban)
  MATLAB Function12/2(c) -> [rol], Scope69/1, Memory8/1
  Memory8/1 -> Switch3/2
  Sum34/1 -> Scope68/1
  Constant24/1 -> Switch3/1
  MATLAB Function12/1(r) -> Sum34/2
  Sum30/1 -> Abs5/1
  Constant28/1 -> Sum35/1
  Constant31/1 -> Switch4/1
  Sum24/1 -> Demux11/1, MATLAB Function13/1(dr)
  Sum35/1 -> Scope51/1
  MATLAB Function13/1(r) -> Sum35/2
  Memory9/1 -> Switch4/2
  Switch4/1 -> MATLAB Function13/2(ban)
  MATLAB Function13/2(c) -> [ruo3], Scope57/1, Memory9/1
  Constant32/1 -> Switch4/3
  Clock2/1 -> MATLAB Function13/3(t)
  Memory10/1 -> Sum36/2
  Memory11/1 -> Sum37/2
  cdis2/1 -> Memory11/1, Sum37/1, Scope87/2, [x_hat_uio12]
  Memory12/1 -> Sum39/2
  Memory13/1 -> Sum40/2
  Abs1/1 -> Memory2/1, Sum24/1, Scope31/1
  Abs/1 -> Memory/1, Sum20/1, Scope25/1
  Abs2/1 -> Memory3/1, Sum25/1, Scope34/1
  Abs3/1 -> Memory4/1, Sum26/1
  Demux1/1 -> Scope77/1
  Demux1/2 -> Scope77/2
  Demux1/3 -> Scope77/3
  Demux1/4 -> Scope77/4
  Sum37/1 -> Demux1/1
  Demux2/1 -> Scope76/1
  Demux2/2 -> Scope76/2
  Demux2/4 -> Scope76/4
  Demux2/3 -> Scope76/3
  Sum36/1 -> Demux2/1
  Demux4/1 -> Scope78/1
  Demux4/2 -> Scope78/2
  Demux4/4 -> Scope78/4
  Demux4/3 -> Scope78/3
  Sum39/1 -> Demux4/1
  Demux9/1 -> Scope79/1
  Demux9/2 -> Scope79/2
  Demux9/4 -> Scope79/4
  Demux9/3 -> Scope79/3
  Sum40/1 -> Demux9/1
  Demux10/1 -> Scope80/1
  Demux10/2 -> Scope80/2
  Demux10/4 -> Scope80/4
  Demux10/3 -> Scope80/3
  Demux11/1 -> Scope81/1
  Demux11/2 -> Scope81/2
  Demux11/4 -> Scope81/4
  Demux11/3 -> Scope81/3
  Demux12/1 -> Scope82/1
  Demux12/2 -> Scope82/2
  Demux12/4 -> Scope82/4
  Demux12/3 -> Scope82/3
  Demux13/1 -> Scope83/1
  Demux13/2 -> Scope83/2
  Demux13/4 -> Scope83/4
  Demux13/3 -> Scope83/3
  Demux14/3 -> Scope33/3
  Demux14/4 -> Delay/1, Scope33/4
  Demux14/2 -> Scope33/2
  Demux14/1 -> Scope33/1
  Abs5/1 -> Demux14/1, MATLAB Function12/1(dr)
  Memory14/1 -> Sum41/2
  Sum41/1 -> Abs4/1
  Abs4/1 -> Scope36/1
  [x_hat_uio3] -> MATLAB Function39/3(x_hat3)
  [x_hat_uio1] -> MATLAB Function38/1(x_hat1)
  [x_hat_uio4] -> MATLAB Function39/4(x_hat4)
  [rol] -> MATLAB Function39/6(rol)
  [x_hat_uio1] -> MATLAB Function39/1(x_hat1)
  [rol] -> MATLAB Function34/6(rol)
  [ruo1] -> MATLAB Function38/5(ruo1)
  [x_hat_uio4] -> MATLAB Function34/4(x_hat4)
  [x_hat_uio1] -> MATLAB Function34/1(x_hat1)
  [x_hat_uio4] -> MATLAB Function38/4(x_hat4)
  [ruo3] -> MATLAB Function39/5(ruo1)
  MATLAB Function34/1(v1) -> [ca2], Sum18/1, Scope53/1
  [x_hat_uio3] -> MATLAB Function34/3(x_hat3)
  [ruo2] -> MATLAB Function34/5(ruo1)
  [x_hat_uio2] -> MATLAB Function34/2(x_hat2)
  [rol] -> MATLAB Function38/6(rol)
  MATLAB Function39/1(v1) -> [ca3], Sum42/1, Scope58/1
  [x_hat_uio2] -> MATLAB Function38/2(x_hat2)
  [x_hat_uio2] -> MATLAB Function39/2(x_hat2)
  [x_hat_uio3] -> MATLAB Function38/3(x_hat3)
  [x_hat_uio21] -> Sum59/1
  [x_hat_uio11] -> Sum58/1
  [x_hat_uio12] -> Sum58/2
  Gain27/1 -> Scope135/1, Scope62/1, [x_hat_uio4]
  [x_hat_uio21] -> Sum60/3
  [x_hat_uio21] -> Sum61/2
  Sum58/1 -> Gain28/1
  [x_hat_uio13] -> Sum59/3
  Gain26/1 -> Scope42/1, Scope60/1, [x_hat_uio3]
  Sum60/1 -> Gain26/1
  [x_hat_uio12] -> Sum61/3
  Gain28/1 -> Scope138/1, [x_hat_uio1]
  [x_hat_uio13] -> Sum58/3
  [x_hat_uio11] -> Sum60/1
  [x_hat_uio13] -> Sum60/2
  Gain29/1 -> Scope59/1, Scope41/1, [x_hat_uio2]
  Sum61/1 -> Gain27/1
  [x_hat_uio11] -> Sum61/1
  [x_hat_uio12] -> Sum59/2
  Sum59/1 -> Gain29/1
  [ruo4] -> MATLAB Function1/5(ruo1)
  [x_hat_uio3] -> MATLAB Function1/3(x_hat3)
  [x_hat_uio1] -> MATLAB Function1/1(x_hat1)
  [x_hat_uio2] -> MATLAB Function1/2(x_hat2)
  [rol] -> MATLAB Function1/6(rol)
  [x_hat_uio4] -> MATLAB Function1/4(x_hat4)
  MeasureNode_I2/2(Out1) -> [a1]
  MeasureNode_I1/2(Out1) -> [a2]
  MeasureNode_I3/2(Out1) -> [a3]
  [a1] -> Sum16/2, Scope109/2
  [a2] -> Sum18/2, Scope53/2
  [a4] -> Sum27/2, Scope52/2
  [a3] -> Sum42/2, Scope58/2
  [x_hat] -> Scope138/2
  [y_ma] -> Scope138/3
  [y_ma] -> Scope59/3
  [x_hat] -> Scope59/2
  [y_ma] -> Scope60/3
  [x_hat] -> Scope60/2
  [y_ma] -> Scope62/3
  [x_hat] -> Scope62/2
  Sum16/1 -> Abs6/1
  Abs6/1 -> [e1], Scope64/1
  Sum18/1 -> Abs7/1
  Abs7/1 -> [e2], Scope70/1
  Sum27/1 -> Abs8/1
  Abs8/1 -> [e4], Scope71/1
  MATLAB Function1/1(v1) -> [ca4], Sum27/1, Scope52/1
  Sum42/1 -> Abs9/1
  Abs9/1 -> [e3], Scope73/1
  Transfer Fcn1/1 -> Scope74/1, Goto1/1
  MeasureNode_I4/2(Out1) -> [a4]
  MeasureNode_I4/1(Out) -> [Vload], [V_vsi]
  MeasureNode_I5/1(Out) -> Goto61/1
  MeasureNode_I5/2(Out1) -> Goto62/1
  [rol] -> Scope84/1
  [ruo4] -> Scope84/5
  [ruo3] -> Scope84/4
  [ruo1] -> Scope84/2
  [ruo2] -> Scope84/3
  Delay/1 -> MATLAB Function12/3(dr1)
  MATLAB Function38/1(v1) -> [ca1], Sum16/1, Scope109/1
  [ca4] -> Scope85/4
  [ca3] -> Scope85/3
  [ca2] -> Scope85/2
  [ca1] -> Scope85/1
  [e4] -> Scope90/4
  [e3] -> Scope90/3
  [e2] -> Scope90/2
  [e1] -> Scope90/1
  CSI_Control_BIO/1(D) -> Scope13/1, Gain15/1
  CSI_Control_BIO1/1(D) -> Gain16/1, Scope20/1
  Sine Wave4/1 -> Sum43/1
  Sum43/1 -> Scope91/1
  [Vload] -> Sum43/2
  Constant15/1 -> LinearProg2/1(P_load), [P_ref]
  Constant17/1 -> [Q_ref], LinearProg3/1(Q_load)

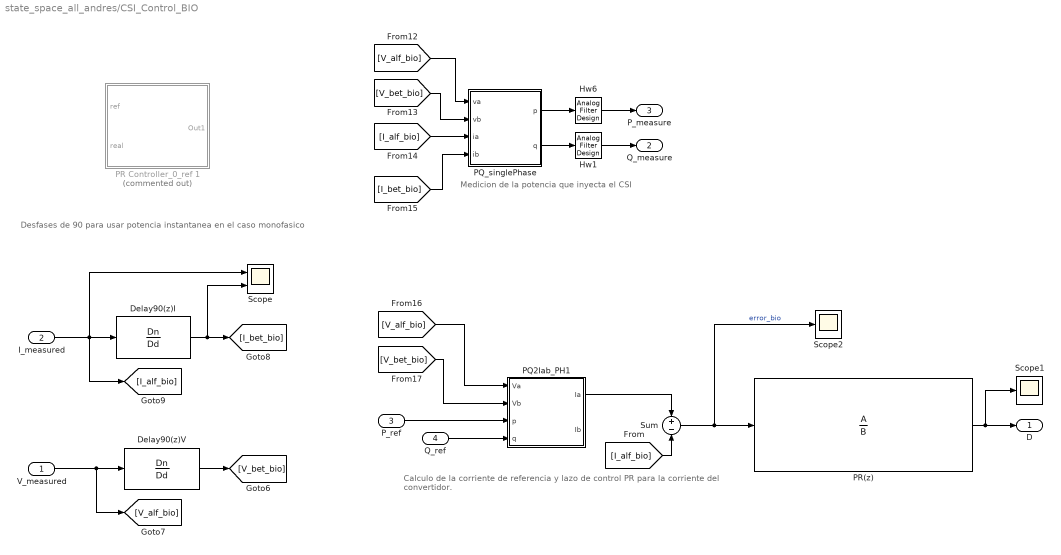
== system state_space_all_andres/CSI_Control_BIO ==
  note: Medicion de la potencia que inyecta el CSI
  note: Desfases de 90 para usar potencia
      | instantanea en el caso monofasico
  note: Calculo de la corriente de referencia
      | y lazo de control PR para la corriente
      | del convertidor.
  V_measured : Inport
  I_measured : Inport  Port=2
  P_ref : Inport  Port=3
  Q_ref : Inport  Port=4
  Delay90(z)I : DiscreteTransferFcn  Numerator=Dn  Denominator=Dd  SampleTime=T
  Delay90(z)V : DiscreteTransferFcn  Numerator=Dn  Denominator=Dd  SampleTime=T
  Hw1 : dsparch4/Analog Filter Design  method=Bessel  filttype=Lowpass  N=4  Wlo=30*2*pi  Whi=80  Rp=2  Rs=80
  Hw6 : dsparch4/Analog Filter Design  method=Bessel  filttype=Lowpass  N=4  Wlo=30*2*pi  Whi=80  Rp=2  Rs=80
  PQ2Iab_PH1 : MATLAB Function  TreatAsAtomicUnit=on
  PQ_singlePhase : MATLAB Function  TreatAsAtomicUnit=on
  PR Controller_0_ref 1 : Subsystem  Commented=on  mask{Kp=40/100, Ki=200, wa=2, w0=60*2*pi, st_time=1e-3}
      mask prompts: Kp "Ganancia Proporcional"; Ki "Ganancia Integral"; wa "Ancho camapana resonancia"; w0 "Frecuencia Central"; st_time "Tiempo muerto (Start)"
      mask Display:
      | port_label('input',1,'ref')
      | port_label('input',2,'sens')
      | port_label('output',1,'out')
      | 
      | plot(.4+[0:.01:pi/10], .32+sin(40*[0:.01:pi/10])/13)
      | 
      | plot([.4 .6],.05+[.5 .7])
      | plot([.4 .6],.05+[.9 .7])
      | plot([.4 .4],.05+[.9 .5])
      | 
      | text(.27,.37,'\fontsize{25} \int', 'texmode', 'on')
  PR(z) : DiscreteTransferFcn  Numerator=A  Denominator=B  SampleTime=T
  Scope : Scope  NumInputPorts=2
  Scope1 : Scope
  Scope2 : Scope
  Sum : Sum  Inputs=+-
  D : Outport
  Q_measure : Outport  Port=2
  P_measure : Outport  Port=3
  wires:
  I_measured/1 -> Scope/1, Delay90(z)I/1, [I_alf_bio]
  [V_bet_bio] -> PQ2Iab_PH1/2(Vb)
  Delay90(z)I/1 -> Scope/2, [I_bet_bio]
  [I_bet_bio] -> PQ_singlePhase/4(ib)
  [I_alf_bio] -> PQ_singlePhase/3(ia)
  [V_alf_bio] -> PQ2Iab_PH1/1(Va)
  Delay90(z)V/1 -> [V_bet_bio]
  [V_bet_bio] -> PQ_singlePhase/2(vb)
  [V_alf_bio] -> PQ_singlePhase/1(va)
  V_measured/1 -> Delay90(z)V/1, [V_alf_bio]
  P_ref/1 -> PQ2Iab_PH1/3(p)
  Q_ref/1 -> PQ2Iab_PH1/4(q)
  Sum/1 -> Scope2/1, PR(z)/1  "error_bio"
  [I_alf_bio] -> Sum/2
  PQ2Iab_PH1/1(Ia) -> Sum/1
  PR(z)/1 -> Scope1/1, D/1
  PQ_singlePhase/2(q) -> Hw1/1
  Hw1/1 -> Q_measure/1
  PQ_singlePhase/1(p) -> Hw6/1
  Hw6/1 -> P_measure/1

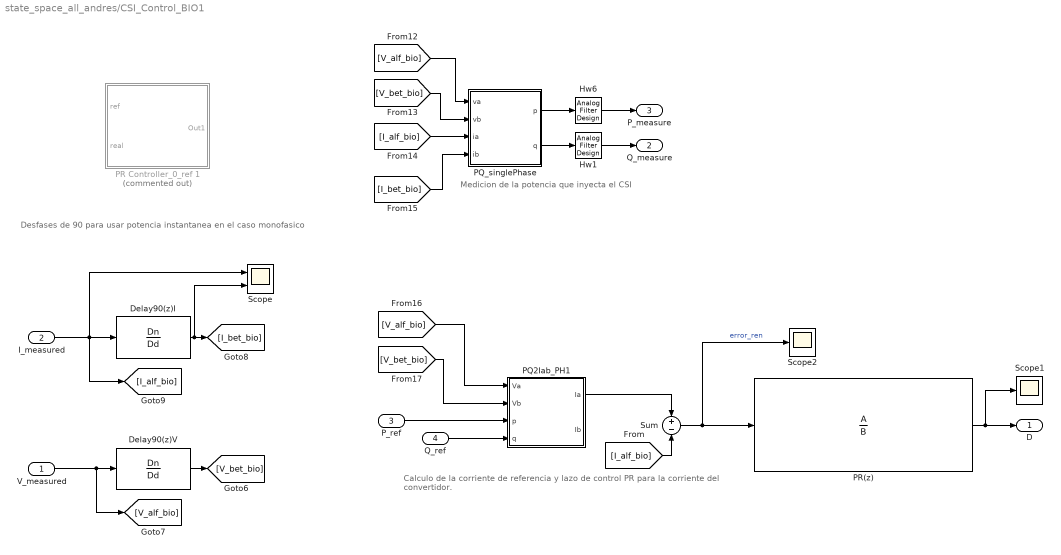
== system state_space_all_andres/CSI_Control_BIO1 ==
  note: Medicion de la potencia que inyecta el CSI
  note: Desfases de 90 para usar potencia
      | instantanea en el caso monofasico
  note: Calculo de la corriente de referencia
      | y lazo de control PR para la corriente
      | del convertidor.
  V_measured : Inport
  I_measured : Inport  Port=2
  P_ref : Inport  Port=3
  Q_ref : Inport  Port=4
  Delay90(z)I : DiscreteTransferFcn  Numerator=Dn  Denominator=Dd  SampleTime=T
  Delay90(z)V : DiscreteTransferFcn  Numerator=Dn  Denominator=Dd  SampleTime=T
  Hw1 : dsparch4/Analog Filter Design  method=Bessel  filttype=Lowpass  N=4  Wlo=30*2*pi  Whi=80  Rp=2  Rs=80
  Hw6 : dsparch4/Analog Filter Design  method=Bessel  filttype=Lowpass  N=4  Wlo=30*2*pi  Whi=80  Rp=2  Rs=80
  PQ2Iab_PH1 : MATLAB Function  TreatAsAtomicUnit=on
  PQ_singlePhase : MATLAB Function  TreatAsAtomicUnit=on
  PR Controller_0_ref 1 : Subsystem  Commented=on  mask{Kp=40/100, Ki=200, wa=2, w0=60*2*pi, st_time=1e-3}
      mask prompts: Kp "Ganancia Proporcional"; Ki "Ganancia Integral"; wa "Ancho camapana resonancia"; w0 "Frecuencia Central"; st_time "Tiempo muerto (Start)"
      mask Display:
      | port_label('input',1,'ref')
      | port_label('input',2,'sens')
      | port_label('output',1,'out')
      | 
      | plot(.4+[0:.01:pi/10], .32+sin(40*[0:.01:pi/10])/13)
      | 
      | plot([.4 .6],.05+[.5 .7])
      | plot([.4 .6],.05+[.9 .7])
      | plot([.4 .4],.05+[.9 .5])
      | 
      | text(.27,.37,'\fontsize{25} \int', 'texmode', 'on')
  PR(z) : DiscreteTransferFcn  Numerator=A  Denominator=B  SampleTime=T
  Scope : Scope  NumInputPorts=2
  Scope1 : Scope
  Scope2 : Scope
  Sum : Sum  Inputs=+-
  D : Outport
  Q_measure : Outport  Port=2
  P_measure : Outport  Port=3
  wires:
  I_measured/1 -> Scope/1, Delay90(z)I/1, [I_alf_bio]
  [V_bet_bio] -> PQ2Iab_PH1/2(Vb)
  Delay90(z)I/1 -> Scope/2, [I_bet_bio]
  [I_bet_bio] -> PQ_singlePhase/4(ib)
  [I_alf_bio] -> PQ_singlePhase/3(ia)
  [V_alf_bio] -> PQ2Iab_PH1/1(Va)
  Delay90(z)V/1 -> [V_bet_bio]
  [V_bet_bio] -> PQ_singlePhase/2(vb)
  [V_alf_bio] -> PQ_singlePhase/1(va)
  V_measured/1 -> Delay90(z)V/1, [V_alf_bio]
  P_ref/1 -> PQ2Iab_PH1/3(p)
  Q_ref/1 -> PQ2Iab_PH1/4(q)
  Sum/1 -> Scope2/1, PR(z)/1  "error_ren"
  [I_alf_bio] -> Sum/2
  PQ2Iab_PH1/1(Ia) -> Sum/1
  PR(z)/1 -> Scope1/1, D/1
  PQ_singlePhase/2(q) -> Hw1/1
  Hw1/1 -> Q_measure/1
  PQ_singlePhase/1(p) -> Hw6/1
  Hw6/1 -> P_measure/1

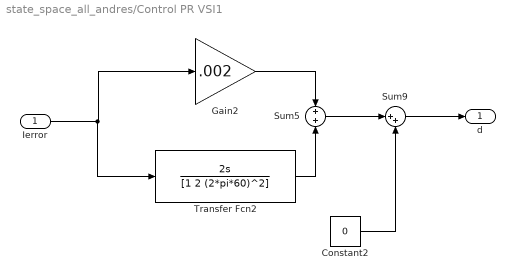
== system state_space_all_andres/Control PR VSI1 ==
  Ierror : Inport
  Constant2 : Constant  Value=0
  Gain2 : Gain  Gain=.002
  Sum5 : Sum  Inputs=+|+
  Sum9 : Sum  Inputs=|++
  Transfer Fcn2 : TransferFcn  Numerator=[2 0]  Denominator=[1 2 (2*pi*60)^2]
  d : Outport
  wires:
  Constant2/1 -> Sum9/2
  Sum5/1 -> Sum9/1
  Transfer Fcn2/1 -> Sum5/2
  Gain2/1 -> Sum5/1
  Ierror/1 -> Transfer Fcn2/1, Gain2/1
  Sum9/1 -> d/1

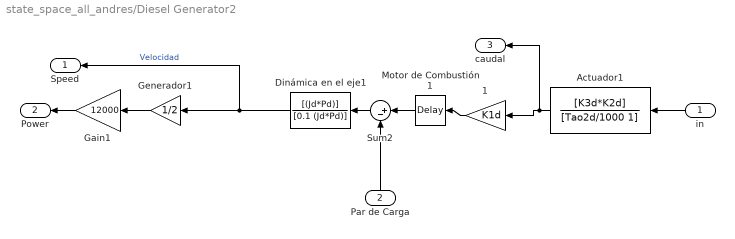
== system state_space_all_andres/Diesel Generator2 ==
  in : Inport
  Par de Carga : Inport  Port=2
  " 1" : Gain  Gain=K1d
  " Generador1" : Gain  Gain=1/2
  Actuador1 : TransferFcn  Numerator=[K3d*K2d]  Denominator=[Tao2d/1000 1]
  Dinámica en el eje1 : TransferFcn  Numerator=[(Jd*Pd)]  Denominator=[0.1 (Jd*Pd)]
  Gain1 : Gain  Gain=12000
  Motor de Combustión1 : TransportDelay  DelayTime=Tao1d
  Sum2 : Sum  Inputs=|+-
  Speed : Outport
  Power : Outport  Port=2
  caudal : Outport  Port=3
  wires:
  " 1"/1 -> Motor de Combustión1/1
  " Generador1"/1 -> Gain1/1
  Motor de Combustión1/1 -> Sum2/1
  Actuador1/1 -> caudal/1, " 1"/1
  Dinámica en el eje1/1 -> Speed/1, " Generador1"/1  "Velocidad"
  Sum2/1 -> Dinámica en el eje1/1
  in/1 -> Actuador1/1
  Par de Carga/1 -> Sum2/2
  Gain1/1 -> Power/1

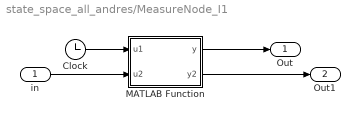
== system state_space_all_andres/MeasureNode_I1 ==
  in : Inport
  Clock : Clock
  MATLAB Function : MATLAB Function  TreatAsAtomicUnit=on
  Out : Outport
  Out1 : Outport  Port=2
  wires:
  MATLAB Function/1(y) -> Out/1
  Clock/1 -> MATLAB Function/1(u1)
  in/1 -> MATLAB Function/2(u2)
  MATLAB Function/2(y2) -> Out1/1

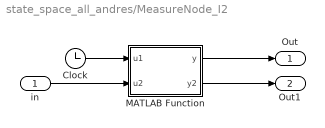
== system state_space_all_andres/MeasureNode_I2 ==
  in : Inport
  Clock : Clock
  MATLAB Function : MATLAB Function  TreatAsAtomicUnit=on
  Out : Outport
  Out1 : Outport  Port=2
  wires:
  MATLAB Function/1(y) -> Out/1
  Clock/1 -> MATLAB Function/1(u1)
  in/1 -> MATLAB Function/2(u2)
  MATLAB Function/2(y2) -> Out1/1

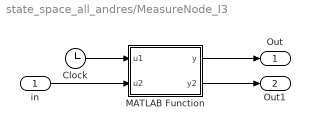
== system state_space_all_andres/MeasureNode_I3 ==
  in : Inport
  Clock : Clock
  MATLAB Function : MATLAB Function  TreatAsAtomicUnit=on
  Out : Outport
  Out1 : Outport  Port=2
  wires:
  MATLAB Function/1(y) -> Out/1
  Clock/1 -> MATLAB Function/1(u1)
  in/1 -> MATLAB Function/2(u2)
  MATLAB Function/2(y2) -> Out1/1

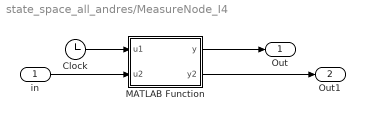
== system state_space_all_andres/MeasureNode_I4 ==
  in : Inport
  Clock : Clock
  MATLAB Function : MATLAB Function  TreatAsAtomicUnit=on
  Out : Outport
  Out1 : Outport  Port=2
  wires:
  MATLAB Function/1(y) -> Out/1
  Clock/1 -> MATLAB Function/1(u1)
  in/1 -> MATLAB Function/2(u2)
  MATLAB Function/2(y2) -> Out1/1

== system state_space_all_andres/MeasureNode_I5 ==
  in : Inport
  Clock : Clock
  MATLAB Function : MATLAB Function  TreatAsAtomicUnit=on
  Out : Outport
  Out1 : Outport  Port=2
  wires:
  MATLAB Function/1(y) -> Out/1
  Clock/1 -> MATLAB Function/1(u1)
  in/1 -> MATLAB Function/2(u2)
  MATLAB Function/2(y2) -> Out1/1
